simulink model "Simulink_Intro_1_24a_Solution"  (R2024a)
settings: Solver=VariableStepAuto  StartTime=0.0  StopTime=10.0  RelTol=1e-3
libraries: simulink x1
settings Model: Creator=nroberts  LastModifiedBy=nroberts

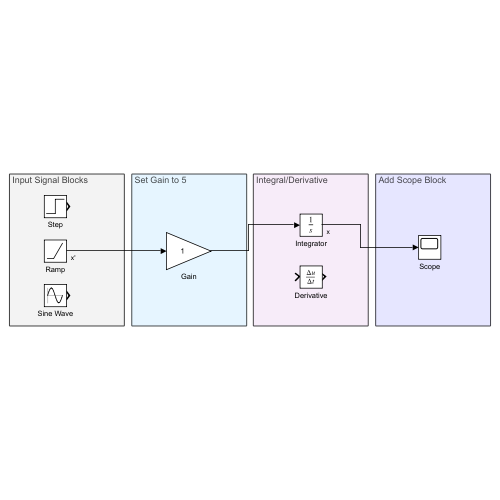
[thumbnail: Simulink's stored preview of the top-level diagram]
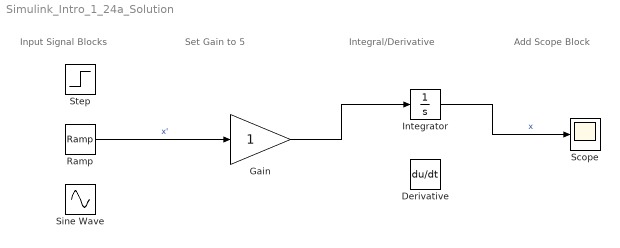
== system Simulink_Intro_1_24a_Solution ==
  note: Add Scope Block
  note: Input Signal Blocks
  note: Set Gain to 5
  note: Integral/Derivative
  Derivative : Derivative
  Gain : Gain
  Integrator : Integrator
  Ramp : simulink/Sources/Ramp  slope=1  start=0  InitialOutput=0
  Scope : Scope
  Sine Wave : Sin  SampleTime=0
  Step : Step  SampleTime=0
  wires:
  Ramp/1 -> Gain/1  "x'"
  Gain/1 -> Integrator/1
  Integrator/1 -> Scope/1  "x"
